simulink model "final_project"  (R2024b)
settings: Solver=FixedStepAuto  StartTime=0.0  StopTime=inf  FixedStep=0.001  RelTol=1e-3  EnableMultiTasking=on
libraries: raspberrypiBasiclib x4
settings Model: ExtModeTrigDuration=2  Creator=gwang  LastModifiedBy=tngusrk
settings SolverCC: PositivePriorityOrder=on
settings OptimizationCC: DefaultParameterBehavior=Inlined  EnhancedBackFolding=on  PassReuseOutputArgsAs=Individual arguments  ZeroExternalMemoryAtStartup=off  ZeroInternalMemoryAtStartup=off  MaxStackSize=200000  OptimizeBlockOrder=speed  DifferentSizesBufferReuse=on  OptimizationCustomize=off  EfficientTunableParamExpr=on
settings DebuggingCC: ParameterTunabilityLossMsg=error
settings HardwareCC: ProdBitPerPointer=32  ProdBitPerSizeT=32  ProdBitPerPtrDiffT=32  ProdLargestAtomicInteger=Long  ProdLargestAtomicFloat=Double  ProdWordSize=32  ProdLongLongMode=on  ProdHWDeviceType=ARM Compatible->ARM Cortex-A (32-bit)  UseEmbeddedCoderFeatures=off
settings RTWCC: Description=Embedded Coder  SystemTargetFile=ert.tlc  HardwareBoard=Raspberry Pi  TLCOptions="-aInlineSetEventsForThisBaseRateFcn=TLC_FALSE -aSuppressMultiTaskScheduler=TLC_FALSE  -aRateBasedStepFcn=0"  TemplateMakefile=ert_default_tmf  Toolchain=GNU GCC Embedded Linux  BuildConfiguration=Specify
settings CodeAppCC: ForceParamTrailComments=on  IgnoreCustomStorageClasses=off  OperatorAnnotations=on  SimulinkDataObjDesc=on  SFDataObjDesc=on  InsertBlockDesc=on
settings ERTTargetCC: SupportNonInlinedSFcns=on  SupportVariableSizeSignals=on  ExtModeTransport=2  ExtModeStaticAlloc=on  ExtModeMexFile=ext_xcp  ExtModeIntrfLevel=Level2 - Open

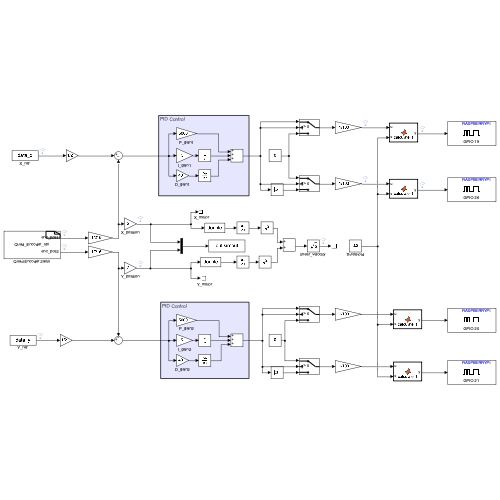
[thumbnail: Simulink's stored preview of the top-level diagram]
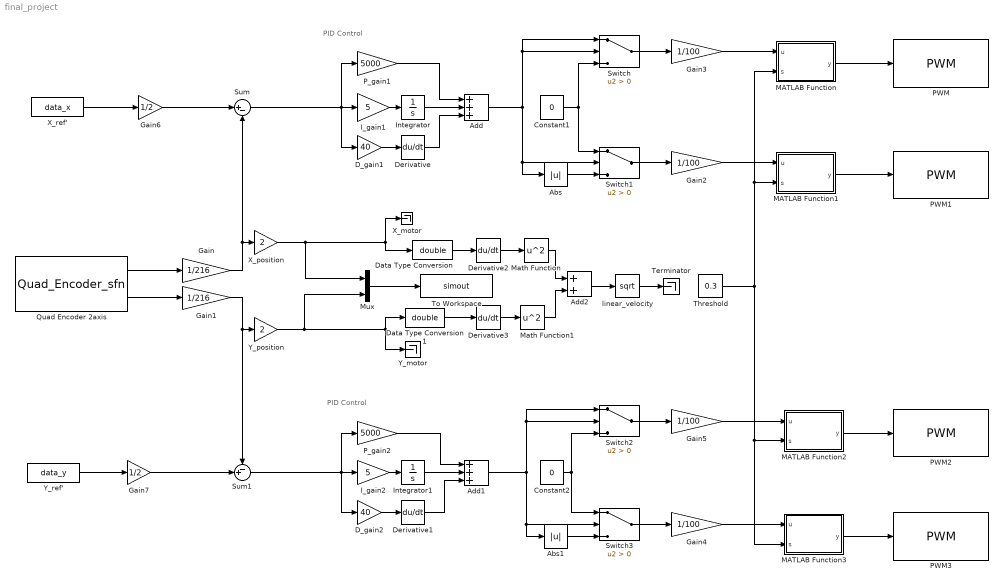
== system final_project ==
  note: PID Control
  note: PID Control
  Abs : Abs  SaturateOnIntegerOverflow=off
  Abs1 : Abs  SaturateOnIntegerOverflow=off
  Add : Sum  Inputs=+++
  Add1 : Sum  Inputs=+++
  Add2 : Sum
  Constant1 : Constant  Value=0
  Constant2 : Constant  Value=0
  D_gain1 : Gain  Gain=40
  D_gain2 : Gain  Gain=40
  Data Type Conversion : DataTypeConversion  OutDataTypeStr=double  SaturateOnIntegerOverflow=off  RndMeth=Floor
  Data Type Conversion1 : DataTypeConversion  OutDataTypeStr=double  SaturateOnIntegerOverflow=off  RndMeth=Floor
  Derivative{,1..3} (4 alike) : Derivative
  Gain : Gain  Gain=1/216
  Gain1 : Gain  Gain=1/216
  Gain{2..5} (4 alike) : Gain  Gain=1/100
  Gain6 : Gain  Gain=1/2
  Gain7 : Gain  Gain=1/2
  I_gain1 : Gain  Gain=5
  I_gain2 : Gain  Gain=5
  Integrator : Integrator
  Integrator1 : Integrator
  MATLAB Function : MATLAB Function  TreatAsAtomicUnit=on
  MATLAB Function1 : MATLAB Function  TreatAsAtomicUnit=on
  MATLAB Function2 : MATLAB Function  TreatAsAtomicUnit=on
  MATLAB Function3 : MATLAB Function  TreatAsAtomicUnit=on
  Math Function : Math  Operator=square
  Math Function1 : Math  Operator=square
  Mux : Mux  Inputs=2
  PWM : raspberrypiBasiclib/PWM  board=Pi 4 Model B  Pin_=19  Frequency=2000  blockPlatform=Raspberry Pi
  PWM1 : raspberrypiBasiclib/PWM  board=Pi 4 Model B  Pin_=26  Frequency=2000  blockPlatform=Raspberry Pi
  PWM2 : raspberrypiBasiclib/PWM  board=Pi 4 Model B  Pin_=20  Frequency=2000  blockPlatform=Raspberry Pi
  PWM3 : raspberrypiBasiclib/PWM  board=Pi 4 Model B  Pin_=21  Frequency=2000  blockPlatform=Raspberry Pi
  P_gain1 : Gain  Gain=5000
  P_gain2 : Gain  Gain=5000
  Quad Encoder 2axis : S-Function  InitFcn=try, set_param(gcb,'FunctionName','Quad_Encoder_sfn'), end  FunctionName=Quad_Encoder_sfn  Parameters=uint8(0),uint8(17),uint8(27),uint8(1),uint8(23),uint8(24)  SFunctionModules=Quad_Encoder_sfn_wrapper.c  SFunctionDeploymentMode=off  EnableBusSupport=off  mask(S-Function Builder){}
      mask init:
      | val = [[.9  0.75 0.75 1 1 .9 .9 1]',[1 1 0.75 0.75 .9 .9 1 .9]'];try , sys = get_param(gcb,'SfunBuilderFcnName');if isempty(sys), sys = get_param(gcb,'FunctionName'); end,catch, sys = get_param(gcb,'FunctionName'); end
      settings: CopyFcn=set_param(gcbh,'LinkStatus','none')  PreSaveFcn=try, set_param(gcb,'FunctionName','Quad_Encoder_sfn'), end  OpenFcn=sfunctionwizard(gcbh)
      mask Display:
      | plot(val(:,1),val(:,2))
      | disp(sys)
      | port_label('output',1,sprintf('%s', 'enc\_pos1'),'interpreter','tex')
      | port_label('output',2,sprintf('%s', 'enc\_pos2'),'interpreter','tex')
  Sum : Sum  Inputs=|+-
  Sum1 : Sum  Inputs=-+|
  Switch{,1..3} (4 alike) : Switch  Criteria=u2 > Threshold  SaturateOnIntegerOverflow=off  InputSameDT=off
  Terminator : Terminator
  Threshold : Constant  Value=0.3
  To Workspace : ToWorkspace  VariableName=simout  SaveFormat=Timeseries  SampleTime=-1
  X_motor : Terminator
  X_position : Gain  Gain=2
  X_ref' : FromWorkspace  VariableName=data_x  OutputAfterFinalValue=Holding final value
  Y_motor : Terminator
  Y_position : Gain  Gain=2
  Y_ref' : FromWorkspace  VariableName=data_y  OutputAfterFinalValue=Holding final value
  linear_velocity : Sqrt
  wires:
  Derivative/1 -> Add/3
  Add/1 -> Abs/1, Switch1/2, Switch/2, Switch/1
  D_gain1/1 -> Derivative/1
  Abs/1 -> Switch1/3
  Gain/1 -> X_position/1, Sum/2
  Switch1/1 -> Gain2/1
  I_gain1/1 -> Integrator/1
  Integrator/1 -> Add/2
  Sum/1 -> P_gain1/1, D_gain1/1, I_gain1/1
  Constant1/1 -> Switch1/1, Switch/3
  P_gain1/1 -> Add/1
  Quad Encoder 2axis/1 -> Gain/1
  Switch/1 -> Gain3/1
  Constant2/1 -> Switch2/3, Switch3/1
  Switch2/1 -> Gain5/1
  Quad Encoder 2axis/2 -> Gain1/1
  P_gain2/1 -> Add1/1
  Switch3/1 -> Gain4/1
  Add1/1 -> Abs1/1, Switch3/2, Switch2/1, Switch2/2
  Integrator1/1 -> Add1/2
  Sum1/1 -> I_gain2/1, D_gain2/1, P_gain2/1
  D_gain2/1 -> Derivative1/1
  I_gain2/1 -> Integrator1/1
  Abs1/1 -> Switch3/3
  Derivative1/1 -> Add1/3
  Gain1/1 -> Y_position/1, Sum1/1
  X_position/1 -> Mux/1, Data Type Conversion/1, X_motor/1
  Y_position/1 -> Mux/2, Data Type Conversion1/1, Y_motor/1
  Math Function1/1 -> Add2/2
  Math Function/1 -> Add2/1
  Add2/1 -> linear_velocity/1
  linear_velocity/1 -> Terminator/1
  Mux/1 -> To Workspace/1
  Derivative2/1 -> Math Function/1
  Derivative3/1 -> Math Function1/1
  Data Type Conversion/1 -> Derivative2/1
  Data Type Conversion1/1 -> Derivative3/1
  Gain7/1 -> Sum1/2
  MATLAB Function/1(y) -> PWM/1
  Gain3/1 -> MATLAB Function/1(u)
  MATLAB Function1/1(y) -> PWM1/1
  Gain6/1 -> Sum/1
  MATLAB Function2/1(y) -> PWM2/1
  MATLAB Function3/1(y) -> PWM3/1
  Gain2/1 -> MATLAB Function1/1(u)
  Gain5/1 -> MATLAB Function2/1(u)
  Gain4/1 -> MATLAB Function3/1(u)
  Threshold/1 -> MATLAB Function2/2(s), MATLAB Function3/2(s), MATLAB Function/2(s), MATLAB Function1/2(s)
  X_ref'/1 -> Gain6/1
  Y_ref'/1 -> Gain7/1

== matlab function final_project/MATLAB Function ==
  data: u input; y output; s input
function y = calculate_f(u, s)

    if u > 1
        y = 1;
    elseif u > s
        y = u;
    elseif u > s/2
        y = s;
    else 
        y = 0;
    end
end

== matlab function final_project/MATLAB Function2 ==
  data: u input; y output; s input
function y = calculate_f(u, s)
% u: 입력 신호
% f: 출력 신호

    if u > 1
        y = 1;
    elseif u > s
        y = u;
    elseif u > s/2
        y = s;
    else % u == 0
        y = 0;
    end
end

== matlab function final_project/MATLAB Function3 ==
  data: u input; y output; s input
function y = calculate_f(u, s)
% u: 입력 신호
% f: 출력 신호

    if u > 1
        y = 1;
    elseif u > s
        y = u;
    elseif u > s/2
        y = s;
    else % u == 0
        y = 0;
    end
end

== matlab function final_project/MATLAB Function1 ==
  data: u input; y output; s input
function y = calculate_f(u, s)
% u: 입력 신호
% f: 출력 신호

    if u > 1
        y = 1;
    elseif u > s
        y = u;
    elseif u > s/2
        y = s;
    else % u == 0
        y = 0;
    end
end
